simulink model "titopSimple_ol"  (Simulink 9.2)
settings: Solver=ode45  StartTime=0.0  StopTime=10.0  RelTol=1e-3
values from neighbouring files (symbols this model uses):
  T21 = [cos(theta2) -sin(theta2) 0; sin(theta2) cos(theta2) 0;0 0 1]    [titopSimple_model.m]    (also in titop_model.m)
undefined symbols (not defined in the file or in its folder): J_payload, m_joint2, m_payload
libraries: cstblocks x2
settings Model: Creator=d.alazard  LastModifiedBy=a.brugnoli
settings DataIOCC: SignalLoggingSaveFormat=Dataset
settings OptimizationCC: BlockReduction=off  BooleanDataType=off
settings DebuggingCC: SaveWithParameterizedLinksMsg=none  SignalResolutionControl=TryResolveAllWithWarning  FcnCallInpInsideContextMsg=error  AllowSymbolicDim=off  StateNameClashWarn=none
settings HardwareCC: TargetUnknown=on
settings GRTTargetCC: CombineOutputUpdateFcns=on  GRTInterface=off
settings ConfigComp: CovSFcnEnable=off

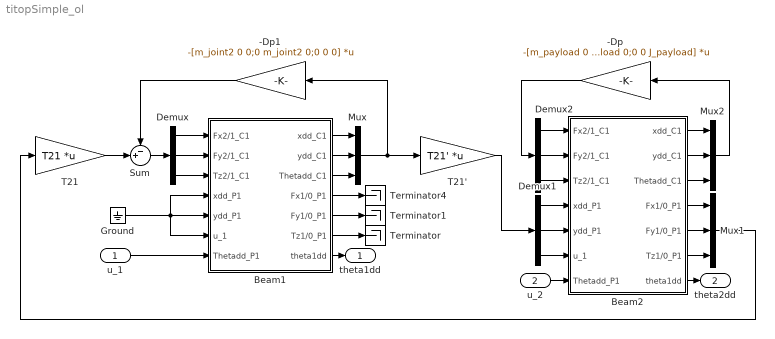
== system titopSimple_ol ==
  u_1 : Inport
  u_2 : Inport  Port=2
  -Dp : Gain  Gain=-[m_payload 0 0;0 m_payload 0;0 0 J_payload]  Multiplication=Matrix(K*u) (u vector)
  -Dp1 : Gain  Gain=-[m_joint2 0 0;0 m_joint2 0;0 0 0]  Multiplication=Matrix(K*u) (u vector)
  Beam1 : Subsystem
  Beam2 : Subsystem
  Demux : Demux  Outputs=3
  Demux1 : Demux  Outputs=3
  Demux2 : Demux  Outputs=3
  Ground : Ground
  Mux : Mux  Inputs=3
  Mux1 : Mux  Inputs=3
  Mux2 : Mux  Inputs=3
  Sum : Sum  Inputs=-+|
  T21 : Gain  Gain=T21  Multiplication=Matrix(K*u) (u vector)
  T21' : Gain  Gain=T21'  Multiplication=Matrix(K*u) (u vector)
  Terminator : Terminator
  Terminator1 : Terminator
  Terminator4 : Terminator
  theta1dd : Outport
  theta2dd : Outport  Port=2
  wires:
  Beam1/4(Fx1/0_P1) -> Terminator4/1
  Beam1/5(Fy1/0_P1) -> Terminator1/1
  Beam1/6(Tz1/0_P1) -> Terminator/1
  Beam1/7(theta1dd) -> theta1dd/1
  Beam1/1(xdd_C1) -> Mux/1
  Beam1/2(ydd_C1) -> Mux/2
  Demux/1 -> Beam1/1(Fx2/1_C1)
  Demux/2 -> Beam1/2(Fy2/1_C1)
  Demux1/1 -> Beam2/4(xdd_P1)
  Demux1/2 -> Beam2/5(ydd_P1)
  Mux/1 -> -Dp1/1, T21'/1
  Beam1/3(Thetadd_C1) -> Mux/3
  Demux/3 -> Beam1/3(Tz2/1_C1)
  Demux1/3 -> Beam2/6(u_1)
  T21'/1 -> Demux1/1
  Mux1/1 -> T21/1
  Mux2/1 -> -Dp/1
  -Dp/1 -> Demux2/1
  u_2/1 -> Beam2/7("Thetadd_P1 ")
  Ground/1 -> Beam1/6(u_1), Beam1/4(xdd_P1), Beam1/5(ydd_P1)
  u_1/1 -> Beam1/7("Thetadd_P1 ")
  Beam2/2(ydd_C1) -> Mux2/2
  Beam2/1(xdd_C1) -> Mux2/1
  Beam2/3(Thetadd_C1) -> Mux2/3
  Beam2/4(Fx1/0_P1) -> Mux1/1
  Beam2/7(theta1dd) -> theta2dd/1
  Beam2/6(Tz1/0_P1) -> Mux1/3
  Beam2/5(Fy1/0_P1) -> Mux1/2
  Demux2/3 -> Beam2/3(Tz2/1_C1)
  Demux2/2 -> Beam2/2(Fy2/1_C1)
  Demux2/1 -> Beam2/1(Fx2/1_C1)
  T21/1 -> Sum/2
  Sum/1 -> Demux/1
  -Dp1/1 -> Sum/1

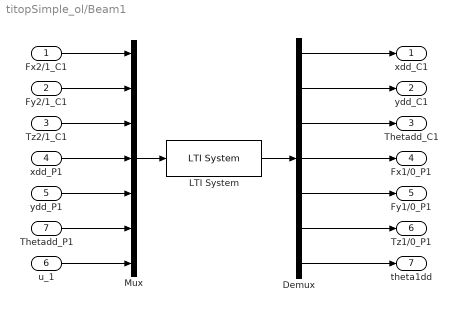
== system titopSimple_ol/Beam1 ==
  Fx2/1_C1 : Inport
  Fy2/1_C1 : Inport  Port=2
  Tz2/1_C1 : Inport  Port=3
  xdd_P1 : Inport  Port=4
  ydd_P1 : Inport  Port=5
  u_1 : Inport  Port=6
  "Thetadd_P1 " : Inport  Port=7
  Demux : Demux  Outputs=7
  LTI System : cstblocks/LTI System  sys=Mbm1_7  IC=[]
  Mux : Mux  Inputs=7
  xdd_C1 : Outport
  ydd_C1 : Outport  Port=2
  Thetadd_C1 : Outport  Port=3
  Fx1/0_P1 : Outport  Port=4
  Fy1/0_P1 : Outport  Port=5
  Tz1/0_P1 : Outport  Port=6
  theta1dd : Outport  Port=7
  wires:
  Fx2/1_C1/1 -> Mux/1
  Fy2/1_C1/1 -> Mux/2
  Tz2/1_C1/1 -> Mux/3
  xdd_P1/1 -> Mux/4
  "Thetadd_P1 "/1 -> Mux/6
  ydd_P1/1 -> Mux/5
  u_1/1 -> Mux/7
  Mux/1 -> LTI System/1
  LTI System/1 -> Demux/1
  Demux/1 -> xdd_C1/1
  Demux/2 -> ydd_C1/1
  Demux/3 -> Thetadd_C1/1
  Demux/4 -> Fx1/0_P1/1
  Demux/5 -> Fy1/0_P1/1
  Demux/6 -> Tz1/0_P1/1
  Demux/7 -> theta1dd/1

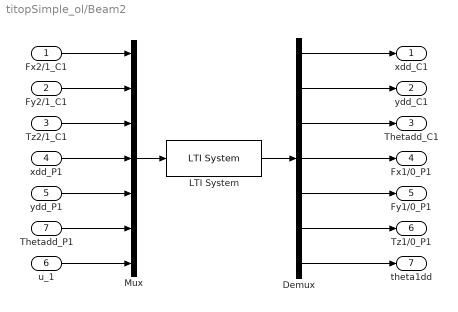
== system titopSimple_ol/Beam2 ==
  Fx2/1_C1 : Inport
  Fy2/1_C1 : Inport  Port=2
  Tz2/1_C1 : Inport  Port=3
  xdd_P1 : Inport  Port=4
  ydd_P1 : Inport  Port=5
  u_1 : Inport  Port=6
  "Thetadd_P1 " : Inport  Port=7
  Demux : Demux  Outputs=7
  LTI System : cstblocks/LTI System  sys=Mbm2_7  IC=[]
  Mux : Mux  Inputs=7
  xdd_C1 : Outport
  ydd_C1 : Outport  Port=2
  Thetadd_C1 : Outport  Port=3
  Fx1/0_P1 : Outport  Port=4
  Fy1/0_P1 : Outport  Port=5
  Tz1/0_P1 : Outport  Port=6
  theta1dd : Outport  Port=7
  wires:
  Tz2/1_C1/1 -> Mux/3
  Fx2/1_C1/1 -> Mux/1
  Demux/2 -> ydd_C1/1
  Demux/7 -> theta1dd/1
  "Thetadd_P1 "/1 -> Mux/6
  Demux/3 -> Thetadd_C1/1
  Demux/1 -> xdd_C1/1
  u_1/1 -> Mux/7
  LTI System/1 -> Demux/1
  Mux/1 -> LTI System/1
  ydd_P1/1 -> Mux/5
  Demux/5 -> Fy1/0_P1/1
  Demux/4 -> Fx1/0_P1/1
  Demux/6 -> Tz1/0_P1/1
  Fy2/1_C1/1 -> Mux/2
  xdd_P1/1 -> Mux/4
